simulink model "idpproject"  (R2021b)
settings: Solver=VariableStepAuto  StartTime=0.0  StopTime=1  RelTol=1e-3
libraries: spsCurrentMeasurementLib x3, spsDCVoltageSourceLib x1, slpidlib x1, spsPermanentMagnetSynchronousMachineLib x1, spsUniversalBridgeLib x1, spspowerguiLib x1
settings Model: Creator=chandu  LastModifiedBy=chandu

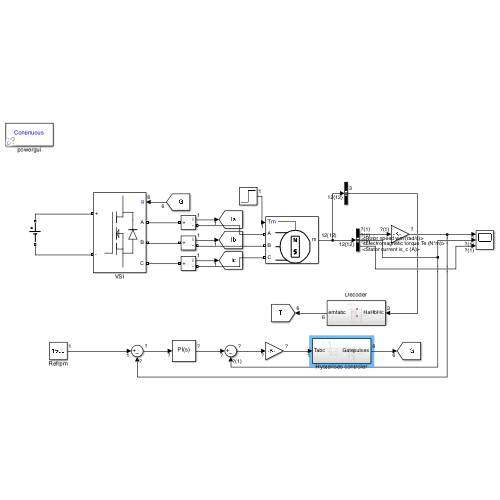
[thumbnail: Simulink's stored preview of the top-level diagram]
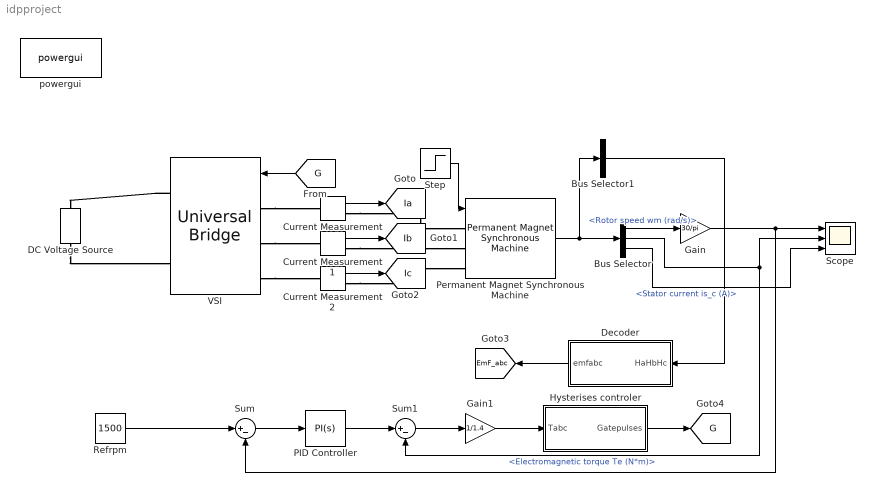
== system idpproject ==
  Bus Selector : BusSelector  OutputSignals=Rotor speed wm (rad/s),Electromagnetic torque Te (N*m),Stator current is_c (A)
  Bus Selector1 : BusSelector  OutputSignals=Hall effect signal h_a,Hall effect signal h_b,Hall effect signal h_c  OutputAsBus=on
  Current Measurement : spsCurrentMeasurementLib/Current Measurement  PhasorSimulation=off  OutputType=Complex  PSBequivalent=0
  Current Measurement1 : spsCurrentMeasurementLib/Current Measurement  PhasorSimulation=off  OutputType=Complex  PSBequivalent=0
  Current Measurement2 : spsCurrentMeasurementLib/Current Measurement  PhasorSimulation=off  OutputType=Complex  PSBequivalent=0
  DC Voltage Source : spsDCVoltageSourceLib/DC Voltage Source  Amplitude=400  Measurements=None
  Decoder : Subsystem
  Gain : Gain  Gain=30/pi
  Gain1 : Gain  Gain=1/1.4
  Hysterises controler : Subsystem
  PID Controller : slpidlib/PID Controller  Controller=PI  Form=Parallel  TimeDomain=Continuous-time  UseExternalTs=off  SampleTime=-1  IntegratorMethod=Forward Euler  FilterMethod=Forward Euler  ControllerParametersSource=internal  P=1  I=1  D=0  UseFilter=on  N=100  TunerSelectOption=Transfer Function Based (PID Tuner App)  InitialConditionSource=internal  InitialConditionForIntegrator=0  InitialConditionForFilter=0  DifferentiatorICPrevScaledInput=0  ExternalReset=none  TrackingMode=off  Kt=1  LimitOutput=off  SatLimitsSource=internal  UpperSaturationLimit=inf  LowerSaturationLimit=-inf  LinearizeAsGain=on  AntiWindupMode=none  Kb=1  POutMin=[]  POutMax=[]  IOutMin=[]  IOutMax=[]  DOutMin=[]  DOutMax=[]  NOutMin=[]  NOutMax=[]  SumOutMin=[]  SumOutMax=[]  SaturationOutMin=[]  SaturationOutMax=[]  PParamMin=[]  PParamMax=[]  IParamMin=[]  IParamMax=[]  DParamMin=[]  DParamMax=[]  NParamMin=[]  NParamMax=[]  KbParamMin=[]  KbParamMax=[]  KtParamMin=[]  KtParamMax=[]  KbOutMin=[]  KbOutMax=[]  KtOutMin=[]  KtOutMax=[]  IntegratorOutMin=[]  IntegratorOutMax=[]  FilterOutMin=[]  FilterOutMax=[]  SumI1OutMin=[]  SumI1OutMax=[]  SumI2OutMin=[]  SumI2OutMax=[]  SumI3OutMin=[]  SumI3OutMax=[]  SumI4OutMin=[]  SumI4OutMax=[]  SumDOutMin=[]  SumDOutMax=[]  DifferentiatorOutMin=[]  DifferentiatorOutMax=[]  FilterDiffOutCoefMin=[]  FilterDiffOutCoefMax=[]  ReciprocalOutMin=[]  ReciprocalOutMax=[]  SumDenOutMin=[]  SumDenOutMax=[]  SumNumOutMin=[]  SumNumOutMax=[]  DivideOutMin=[]  DivideOutMax=[]  UdiffTsProdOutMin=[]  UdiffTsProdOutMax=[]  NTsProdOutMin=[]  NTsProdOutMax=[]  UintegralTsProdOutMin=[]  UintegralTsProdOutMax=[]  UngainTsProdOutMin=[]  UngainTsProdOutMax=[]  IntegratorContinuousStateAttributes=''  IntegratorStateMustResolveToSignalObject=off  IntegratorRTWStateStorageClass=Auto  FilterContinuousStateAttributes=''  FilterStateMustResolveToSignalObject=off  FilterRTWStateStorageClass=Auto  ParallelPVariant=InternalParameters  IdealPVariant=Disabled  IVariant=InternalParameters  DVariant=Disabled  IntegratorVariant=Continuous  SatVariant=Disabled  AWVariant=Passthrough  PCopyVariant=Disabled  TRVariant=Disabled  FdbkBlocksVariant=Forward  IdealPFdbkVariant=Disabled  SatFdbkVariant=Disabled  DerivativeFilterVariant=Disabled  NVariant=Disabled  NCopyVariant=Disabled_SignalSpec  FilterICVariant=Disabled  IntegratorICVariant=InternalICs  ExternalResetVariant=Disabled  TRSumVariant=Passthrough  SumFdbkVariant=Disabled  SumVariant=Sum_PI  TsampFilterVariant=InternalTs  TsampNgainVariant=Passthrough  TsampIntegralVariant=Passthrough  ExternalSaturationOutDataTypeStr=Inherit: Same as second input
  Permanent Magnet Synchronous Machine : spsPermanentMagnetSynchronousMachineLib/Permanent Magnet Synchronous Machine  NbPhases=3  FluxDistribution=Trapezoidal  RotorType=Round  MechanicalLoad=Torque Tm  PresetModel=No  ShowDetailedParameters=on  MeasurementBus=off  Resistance=0.0485  Inductance=8.5e-3  dqInductances=[8.5e-3,8.5e-3]  La=0.000395  MachineConstant=Flux linkage established by magnets (V.s)  Flux=0.1194  VoltageCst=100.0283  TorqueCst=0.9552  Flat=120  Mechanical=[0.0027 0.0004924 4 0]  PolePairs=4  InitialConditions=[0,0, 0,0]  InitialConditions5ph=[0 0 0 0 0 0]  RefAngle=90 degrees behind phase A axis (modified Park)  IterativeDiscreteModel=Trapezoidal non iterative  TsBlock=-1  TsPowergui=0
  Refrpm : Constant  Value=1500
  Scope : Scope  NumInputPorts=3
  Step : Step  SampleTime=0
  Sum : Sum  Inputs=|+-
  Sum1 : Sum  Inputs=|+-
  VSI : spsUniversalBridgeLib/Universal Bridge  Arms=3  SnubberResistance=5000  SnubberCapacitance=1e-6  Device=MOSFET / Diodes  Ron=1e-3  Lon=0  ForwardVoltages="[  0  0  ]"  ForwardVoltage=0  GTOparameters=[ 10e-6 , 20e-6 ]  IGBTparameters=[ 1e-6 , 2e-6 ]  Measurements=None  Measurements_2=None  converterType=Rectifier
  powergui : spspowerguiLib/powergui  Priority=1  SimulationMode=Continuous  SampleTime=50e-6  frequency=60  Iterations=50  frequencyindice=0  Pbase=100e6  ErrMax=1e-4  UnitsV=kV  UnitsW=MW  buscounter=0  FunctionMessages=off  echomessages=off  EnableUseOfTLC=off  CurrentSourceSwitches=off  DisableSnubberDevices=off  DisableRonSwitches=off  DisableVfSwitches=off  DisplayEquations=off  AutomaticDiscreteSolvers=off  SolverType=Tustin/Backward Euler (TBE)  Interpol=off  ExternalGateDelay=off  methode=off  Ts=100  x0status=blocks  SPID=on  SwTol=0  HookPort=off  NonlinearTolerance=1e-4  nMaxIteration=100  ContinueOnMaxIteration=off  RestoreLinks=warning  ResistiveCurrentMeasurement=off  Frange=[0:2:500]  Ylog=off  Xlog=on  ShowGrid=off  save=off  variable=ZData  structure=0  ZoomFFT=off  StartTime=0.0  cycles=1  DisplayStyle=1  fundamental=60  FreqAxis=off  MaxFrequency=1000  frequencyindicesteady=1  RmsSteady=1  display=off
  tag scope: EmF_abc=global, G=global, Ia=global, Ib=global, Ic=global
  wires:
  Step/1 -> Permanent Magnet Synchronous Machine/1
  Current Measurement/1 -> [Ia]
  Current Measurement1/1 -> [Ib]
  Current Measurement2/1 -> [Ic]
  Permanent Magnet Synchronous Machine/1 -> Bus Selector1/1, Bus Selector/1
  Bus Selector/1 -> Gain/1  "<Rotor speed wm (rad/s)>"
  Gain/1 -> Scope/1, Sum/2
  Bus Selector/2 -> Sum1/2, Scope/2  "<Electromagnetic torque Te (N*m)>"
  Bus Selector/3 -> Scope/3  "<Stator current is_c (A)>"
  Bus Selector1/1 -> Decoder/1(HaHbHc)
  Decoder/1(emfabc) -> [EmF_abc]
  Refrpm/1 -> Sum/1
  Sum/1 -> PID Controller/1
  PID Controller/1 -> Sum1/1
  Sum1/1 -> Gain1/1
  Gain1/1 -> Hysterises controler/1(Tabc)
  Hysterises controler/1(Gatepulses) -> [G]
  [G] -> VSI/1
  connections:
  VSI/RConn1 -- DC Voltage Source/RConn1
  DC Voltage Source/LConn1 -- VSI/RConn2
  VSI/LConn1 -- Current Measurement/LConn1
  VSI/LConn2 -- Current Measurement1/LConn1
  VSI/LConn3 -- Current Measurement2/LConn1
  Current Measurement/RConn1 -- Permanent Magnet Synchronous Machine/LConn1
  Current Measurement1/RConn1 -- Permanent Magnet Synchronous Machine/LConn2
  Current Measurement2/RConn1 -- Permanent Magnet Synchronous Machine/LConn3

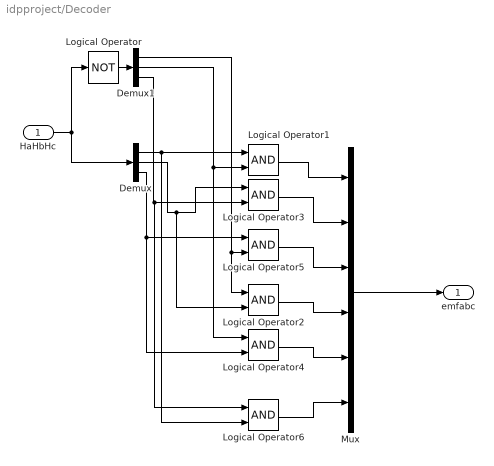
== system idpproject/Decoder ==
  HaHbHc : Inport
  Demux : Demux  Outputs=3
  Demux1 : Demux  Outputs=3
  Logical Operator : Logic  Operator=NOT  AllPortsSameDT=off  OutDataTypeStr=boolean
  Logical Operator{1..6} (6 alike) : Logic  AllPortsSameDT=off  OutDataTypeStr=boolean
  Mux : Mux  Inputs=6
  emfabc : Outport
  wires:
  HaHbHc/1 -> Logical Operator/1, Demux/1
  Logical Operator/1 -> Demux1/1
  Demux/2 -> Logical Operator3/1, Logical Operator2/2
  Demux1/1 -> Logical Operator5/2, Logical Operator2/1
  Demux1/3 -> Logical Operator6/1, Logical Operator3/2
  Demux1/2 -> Logical Operator4/1, Logical Operator1/2
  Demux/3 -> Logical Operator5/1, Logical Operator4/2
  Demux/1 -> Logical Operator6/2, Logical Operator1/1
  Logical Operator1/1 -> Mux/1
  Logical Operator3/1 -> Mux/2
  Logical Operator5/1 -> Mux/3
  Logical Operator2/1 -> Mux/4
  Logical Operator4/1 -> Mux/5
  Logical Operator6/1 -> Mux/6
  Mux/1 -> emfabc/1

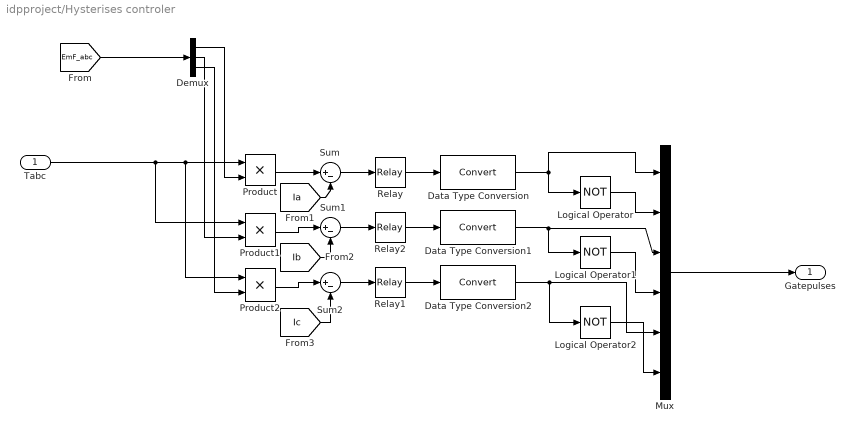
== system idpproject/Hysterises controler ==
  Tabc : Inport
  Data Type Conversion : DataTypeConversion
  Data Type Conversion1 : DataTypeConversion
  Data Type Conversion2 : DataTypeConversion
  Demux : Demux  Outputs=3
  Logical Operator : Logic  Operator=NOT  AllPortsSameDT=off  OutDataTypeStr=boolean
  Logical Operator1 : Logic  Operator=NOT  AllPortsSameDT=off  OutDataTypeStr=boolean
  Logical Operator2 : Logic  Operator=NOT  AllPortsSameDT=off  OutDataTypeStr=boolean
  Mux : Mux  Inputs=6
  Product : Product
  Product1 : Product
  Product2 : Product
  Relay : Relay
  Relay1 : Relay
  Relay2 : Relay
  Sum : Sum  Inputs=|+-
  Sum1 : Sum  Inputs=|+-
  Sum2 : Sum  Inputs=|+-
  Gatepulses : Outport
  wires:
  [EmF_abc] -> Demux/1
  Tabc/1 -> Product1/1, Product2/1, Product/1
  Demux/1 -> Product/2
  Product/1 -> Sum/1
  Product1/1 -> Sum1/1
  Product2/1 -> Sum2/1
  [Ia] -> Sum/2
  [Ib] -> Sum1/2
  [Ic] -> Sum2/2
  Sum/1 -> Relay/1
  Sum1/1 -> Relay2/1
  Sum2/1 -> Relay1/1
  Relay2/1 -> Data Type Conversion1/1
  Relay/1 -> Data Type Conversion/1
  Relay1/1 -> Data Type Conversion2/1
  Data Type Conversion1/1 -> Mux/3, Logical Operator1/1
  Data Type Conversion/1 -> Mux/1, Logical Operator/1
  Logical Operator/1 -> Mux/2
  Logical Operator1/1 -> Mux/4
  Logical Operator2/1 -> Mux/6
  Data Type Conversion2/1 -> Logical Operator2/1, Mux/5
  Mux/1 -> Gatepulses/1
  Demux/2 -> Product1/2
  Demux/3 -> Product2/2
